simulink model "CD_SIMULINK"  (R2023b)
settings: Solver=VariableStepAuto  StartTime=0.0  StopTime=.01  RelTol=1e-3
values from neighbouring files (symbols this model uses):
  C = 10e-6    (= 1e-05)    [CD.m]    (also in Parametros_CD.m)
  d = 0.381    [CD.m]    (also in Parametros_CD.m)
  L = 2e-3    (= 0.002)    [CD.m]    (also in Parametros_CD.m)
  R = 10    [CD.m]    (also in Parametros_CD.m)
  U = 32    [CD.m]    (also in Parametros_CD.m)
settings Model: Creator=User  LastModifiedBy=mluser

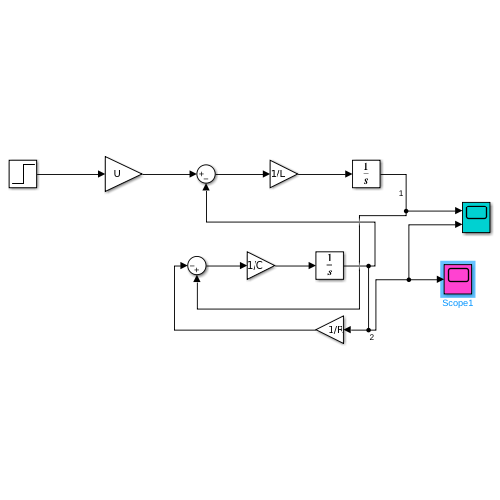
[thumbnail: Simulink's stored preview of the top-level diagram]
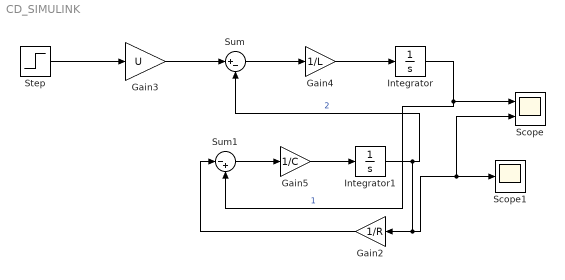
== system CD_SIMULINK ==
  Gain2 : Gain  Gain=1/R
  Gain3 : Gain  Gain=U
  Gain4 : Gain  Gain=1/L
  Gain5 : Gain  Gain=1/C
  Integrator : Integrator
  Integrator1 : Integrator
  Scope : Scope  NumInputPorts=2
  Scope1 : Scope
  Step : Step  Time=0  After=d  SampleTime=0
  Sum : Sum  Inputs=|+-
  Sum1 : Sum  Inputs=|-+
  wires:
  Step/1 -> Gain3/1
  Sum/1 -> Gain4/1
  Gain4/1 -> Integrator/1
  Gain3/1 -> Sum/1
  Integrator1/1 -> Sum/2, Scope/2, Scope1/1, Gain2/1  "2"
  Gain2/1 -> Sum1/1
  Gain5/1 -> Integrator1/1
  Sum1/1 -> Gain5/1
  Integrator/1 -> Sum1/2, Scope/1  "1"
